simulink model "Demo_Kinect"  (R2014a)
settings: Solver=FixedStepDiscrete  SolverMode=SingleTasking  StartTime=0.0  StopTime=inf  FixedStep=0.01  RelTol=1e-3
PostLoadFcn:
  | h_RPStest = RPStest;
model workspace (MAT data in the model file):
  gtest = 0
undefined symbols (not defined in the file or in its folder): avert, avert_gaze_dirs_chance, avert_gaze_duration_factor, avert_head_frequency_factor, avert_head_speed, BML, BML1, BML2, bmlsL, bmlsM, bodyBusyFlag, clock, emotion_amount_factor, faceBusyFlag, fileID, GAZE_WIN, gazing, mutual_gaze_duration_factor, P, pose_chanc_factor, pose_chance_factor, pose_change_flag, pose_frequency_factor, pose_lean, pose_lean_flag, pose_selfAdaptor_chance_factor, pose_speed, pr, serial, STATE_BEFORE, STATE_GO, STATE_OVER, STATE_READY, Stateflow
libraries: simulink x22, instrumentlib x6, lib_affectiveChar_behavior x3, realtime_pacer_lib x2, lib_affectiveChar_input x1
(part 1 of 7)
CloseFcn:
  | % Try to close the GUI
  | % The user might have already closed it.
  | try
  | close(h_RPStest)
  | end
settings Model: ExtModeTrigDuration=2  Creator=Ulysses  LastModifiedBy=root180
settings OptimizationCC: OptimizeModelRefInitCode=on  LifeSpan=1
settings DebuggingCC: UnderspecifiedInitializationDetection=Classic  SolverPrmCheckMsg=none
settings HardwareCC: ProdBitPerInt=16  ProdBitPerPointer=8  ProdIntDivRoundTo=Zero  ProdEndianess=LittleEndian  ProdWordSize=8  ProdHWDeviceType=Atmel->AVR
settings RTWCC: SystemTargetFile=realtime.tlc  GenerateMakefile=off  TemplateMakefile=realtime.tmf  Description=Run on Target Hardware  RTWVerbose=off  ProcessScript=realtime_make_rtw_hook
settings STFCustomTargetCC: TargetLibSuffix=.a  GenerateSampleERTMain=on  ConcurrentExecutionCompliant=off  GeneratePreprocessorConditionals=Use local settings  ERTCustomFileBanners=on  SupportNonInlinedSFcns=off  SupportVariableSizeSignals=on  MATLABClassNameForMDSCustomization=Simulink.SoftwareTarget.ERTCustomization  GRTInterface=off  SystemTargetFile=realtime.tlc
settings ERTTargetCC: CombineOutputUpdateFcns=off  SupportContinuousTime=on  SupportVariableSizeSignals=on  ExtModeTransport=3  ExtModeMexFile=ext_serial_win32_comm  ExtModeMexArgs=0 1 9600  ERTSrcFileBannerTemplate=realtime_code_template.cgt  ERTHdrFileBannerTemplate=realtime_code_template.cgt  ERTDataSrcFileTemplate=realtime_code_template.cgt  ERTDataHdrFileTemplate=realtime_code_template.cgt  ERTCustomFileTemplate=realtime_file_process.tlc

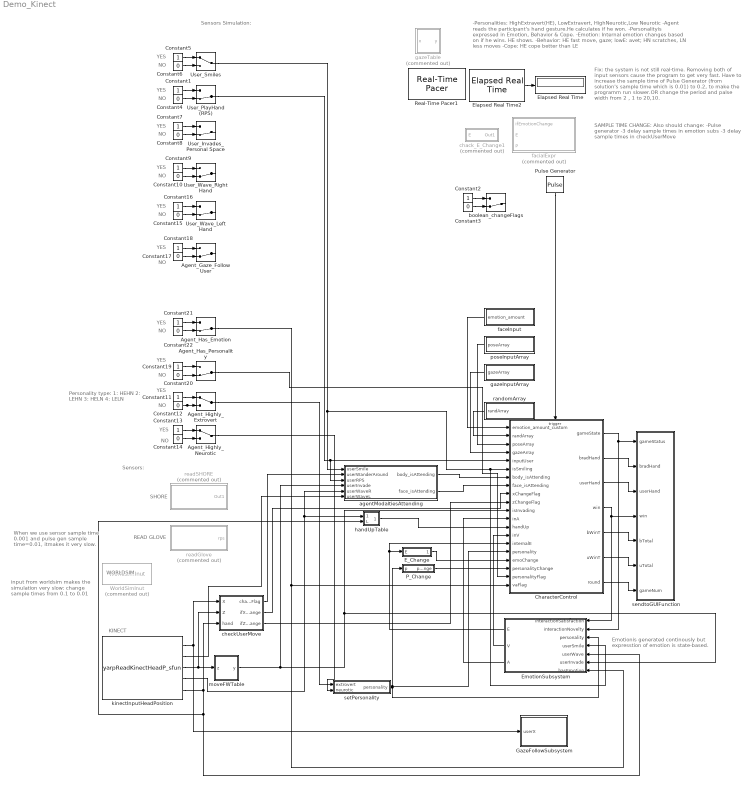
== system Demo_Kinect ==
  note: Sensors Simulation:
  note: YES
  note: YES
  note: Emotionis generated continously but expresstion of emotion is state-based.
  note: WORLDSIM
  note: SHORE
  note: READ GLOVE
  note: SAMPLE TIME CHANGE:
      | Also should change:
      | -Pulse generator
      | -3 delay sample times in emotion subs
      | -3 delay sample times in checkUserMove
  note: When we use sensor sample time 0.001 and pulse gen sample time=0.01, itmakes it very slow.
  note: input from worldsim makes the simulation very slow: change sample times from 0.1 to 0.01
  note: -Personalities: HighExtravert(HE), LowExtravert, HighNeurotic,Low Neurotic
      | -Agent reads the participant's hand gesture.He  calculates if he won.
      | -Personalityis expressed in Emotion, Behavior & Cope.
      | -Emotion: Internal emotion changes based on if he wins. HE shows.
      | -Behavior: HE fast move, gaze; lowE: avet; HN scratches, LN less moves
      | -Cope: HE cope better than LE
  note: Fix: the system is not still real-time. Removing both of input sensors cause the program to get very fast. Have to increase the sample time of Pulse Generator (from solution's sample time which is 0.01) to 0.2, to make the programm run slower.OR change the period and palse width from 2 , 1 to 20,10.
  note: YES
  note: YES
  note: YES
  note: YES
  note: YES
  note: NO
  note: NO
  note: NO
  note: NO
  note: NO
  note: NO
  note: NO
  note: YES
  note: NO
  note: Personality type:
      | 1: HEHN
      | 2: LEHN
      | 3: HELN
      | 4: LELN
  note: Sensors:
  note: KINECT
  note: YES
  note: NO
  note: YES
  note: NO
  Agent_Gaze_Follow User : ManualSwitch  CurrentSetting=0
  Agent_Has_Emotion : ManualSwitch  CurrentSetting=0
  Agent_Has_Personality : ManualSwitch  CurrentSetting=0
  Agent_Highly_Extrovert : ManualSwitch
  Agent_Highly_Neurotic : ManualSwitch
  CharacterControl : Stateflow chart  TreatAsAtomicUnit=on
  Constant{1,5,7,9,16,18} (6 alike) : Constant  OutDataTypeStr=double
  Constant{4,6,8,10,15,17} (6 alike) : Constant  Value=0  OutDataTypeStr=double
  Constant{2,11,13,19,21} (5 alike) : Constant  OutDataTypeStr=boolean
  Constant{3,12,14,20,22} (5 alike) : Constant  Value=0  OutDataTypeStr=boolean
  E_Change : Subsystem
  Elapsed Real Time : Display
      settings: Decimation=2
  Elapsed Real Time2 : realtime_pacer_lib/Elapsed Real Time
  EmotionSubsystem : Subsystem
  GazeFollowSubsystem : Subsystem
  P_Change : Subsystem
  Pulse Generator : DiscretePulseGenerator  SampleTime=0.01
  Real-Time Pacer1 : realtime_pacer_lib/Real-Time Pacer  simTimePerRealTime=1
  User_Invades_Personal Space : ManualSwitch  CurrentSetting=0
  User_PlayHand (RPS) : ManualSwitch  CurrentSetting=0
  User_Smiles : ManualSwitch
  User_Wave_Left Hand : ManualSwitch  CurrentSetting=0
  User_Wave_Right Hand : ManualSwitch  CurrentSetting=0
  WorldSimInut : lib_affectiveChar_input/WorldSimInut  Commented=on
  agentModaltiesAttending : Subsystem
  boolean_changeFlags : ManualSwitch  CurrentSetting=0
  chack_E_Change1 : Subsystem  Commented=on
  checkUserMove : Subsystem
  faceInput : Subsystem
  facialExpr : Subsystem  Commented=on
  gazeInputArray : Subsystem
  gazeTable : Truth Table  Commented=on  TreatAsAtomicUnit=on
  handUpTable : Truth Table  TreatAsAtomicUnit=on
  kinectInputHeadPosition : M-S-Function  FunctionName=yarpReadKinectHeadP_sfun  Parameters='/mary/output','/simulink/in0'
  moveFWTable : Truth Table  TreatAsAtomicUnit=on
  poseInputArray : Subsystem
  randomArray : Subsystem
  readGlove : Subsystem  Commented=on  AncestorBlock=lib_affectiveChar_input/readGlove
  readSHORE : Subsystem  Commented=on  AncestorBlock=lib_affectiveChar_input/readSHORE
  sendtoGUIFunction : MATLAB Function  TreatAsAtomicUnit=on
  setPersonality : MATLAB Function  TreatAsAtomicUnit=on
  wires:
  CharacterControl/1(gameState) -> EmotionSubsystem/2(interactionNovelty), sendtoGUIFunction/1(gameStatus)
  CharacterControl/2(bradHand) -> sendtoGUIFunction/2(bradHand)
  CharacterControl/3(userHand) -> sendtoGUIFunction/3(userHand)
  CharacterControl/6(uWinT) -> sendtoGUIFunction/6(uTotal)
  CharacterControl/7(round) -> sendtoGUIFunction/7(gameNum)
  kinectInputHeadPosition/3 -> moveFWTable/1(z), checkUserMove/2(Z)
  Elapsed Real Time2/1 -> Elapsed Real Time/1
  Pulse Generator/1 -> CharacterControl/Trigger
  CharacterControl/5(bWinT) -> sendtoGUIFunction/5(bTotal)
  CharacterControl/4(win) -> EmotionSubsystem/1(interactionSatisfaction), sendtoGUIFunction/4(win)
  kinectInputHeadPosition/5 -> handUpTable/2(L), EmotionSubsystem/5(userWave), checkUserMove/3(hand)
  kinectInputHeadPosition/1 -> checkUserMove/1(X), GazeFollowSubsystem/1(userX)
  randomArray/1(randArray) -> CharacterControl/2(randArray)
  EmotionSubsystem/1(E) -> CharacterControl/15(internalE), E_Change/1(E)
  EmotionSubsystem/2(V) -> CharacterControl/14(inV)
  EmotionSubsystem/3(A) -> CharacterControl/12(inA)
  E_Change/1(eChange) -> CharacterControl/17(emoChange)
  Constant8/1 -> User_Invades_Personal Space/2
  Constant7/1 -> User_Invades_Personal Space/1
  Constant10/1 -> User_Wave_Right Hand/2
  Constant9/1 -> User_Wave_Right Hand/1
  Constant12/1 -> Agent_Highly_Extrovert/2
  Constant11/1 -> Agent_Highly_Extrovert/1
  Constant14/1 -> Agent_Highly_Neurotic/2
  Constant13/1 -> Agent_Highly_Neurotic/1
  Agent_Highly_Extrovert/1 -> setPersonality/1(extrovert)
  Agent_Highly_Neurotic/1 -> setPersonality/2(neurotic)
  setPersonality/1(personality) -> EmotionSubsystem/3(personality), P_Change/1(p), CharacterControl/16(personality)
  Constant3/1 -> boolean_changeFlags/2
  Constant2/1 -> boolean_changeFlags/1
  Constant4/1 -> User_PlayHand (RPS)/2
  Constant1/1 -> User_PlayHand (RPS)/1
  Constant6/1 -> User_Smiles/2
  Constant5/1 -> User_Smiles/1
  User_PlayHand (RPS)/1 -> CharacterControl/5(inputUser), agentModaltiesAttending/3(userRPS)
  User_Smiles/1 -> agentModaltiesAttending/1(userSmile), CharacterControl/6(isSmiling), EmotionSubsystem/4(userSmile)
  P_Change/1(pChange) -> CharacterControl/18(personalityChange)
  Constant15/1 -> User_Wave_Left Hand/2
  Constant16/1 -> User_Wave_Left Hand/1
  Constant17/1 -> Agent_Gaze_Follow User/2
  Constant18/1 -> Agent_Gaze_Follow User/1
  gazeInputArray/1(gazeArray) -> CharacterControl/4(gazeArray)
  Constant19/1 -> Agent_Has_Personality/1
  Constant20/1 -> Agent_Has_Personality/2
  Constant21/1 -> Agent_Has_Emotion/1
  Constant22/1 -> Agent_Has_Emotion/2
  Agent_Has_Emotion/1 -> EmotionSubsystem/7(hasEmotion), CharacterControl/20(vaFlag)
  Agent_Has_Personality/1 -> CharacterControl/19(personalityFlag)
  poseInputArray/1(poseArray) -> CharacterControl/3(poseArray)
  faceInput/1(emotion_amount) -> CharacterControl/1(emotion_amount_custom)
  moveFWTable/1(y) -> agentModaltiesAttending/4(userInvade), EmotionSubsystem/6(userInvade), CharacterControl/11(isInvading)
  checkUserMove/2(ifXChange) -> CharacterControl/9(xChangeFlag)
  checkUserMove/3(ifZChange) -> CharacterControl/10(zChangeFlag)
  agentModaltiesAttending/1(body_isAttending) -> CharacterControl/7(body_isAttending)
  agentModaltiesAttending/2(face_isAttending) -> CharacterControl/8(face_isAttending)
  kinectInputHeadPosition/4 -> handUpTable/1(R), agentModaltiesAttending/5(userWaveR)
  kinectInputHeadPosition/2 -> agentModaltiesAttending/6(userWaveL)
  handUpTable/1(y) -> CharacterControl/13(handUp)
  checkUserMove/1(changeFlag) -> agentModaltiesAttending/2(userWanderAround)

== system Demo_Kinect/CharacterControl/Gaze_Controller ==
  randArray : Inport
  personality : Inport  Port=2
  inV : Inport  Port=3
  inA : Inport  Port=4
  personalityChange : Inport  Port=5
  gazeArray : Inport  Port=6
  secs : TriggerPort  ShowOutputPort=on
  " Demux " : Demux  Outputs=1
  " SFunction " : S-Function  Tag=Stateflow S-Function Demo_KinectWaveWalkInvade 9  FunctionName=sf_sfun  PortCounts=[7 2]  EnableBusSupport=off
  " Terminator " : Terminator
  gameState : Outport
  wires:
  randArray/1 -> " SFunction "/1
  personality/1 -> " SFunction "/2
  inV/1 -> " SFunction "/3
  inA/1 -> " SFunction "/4
  personalityChange/1 -> " SFunction "/5
  gazeArray/1 -> " SFunction "/6
  " SFunction "/2 -> gameState/1  "gameState"
  " Demux "/1 -> " Terminator "/1
  secs/1 -> " SFunction "/7
  " SFunction "/1 -> " Demux "/1

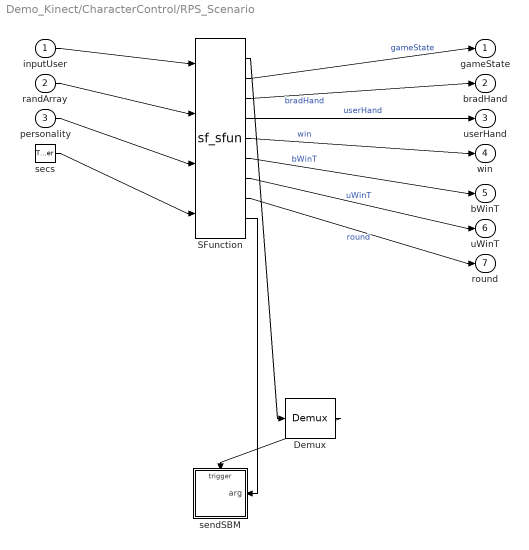
== system Demo_Kinect/CharacterControl/RPS_Scenario ==
  inputUser : Inport
  randArray : Inport  Port=2
  personality : Inport  Port=3
  secs : TriggerPort  ShowOutputPort=on
  " Demux " : Demux  Outputs=1
  " SFunction " : S-Function  Tag=Stateflow S-Function Demo_KinectWaveWalkInvade 5  FunctionName=sf_sfun  PortCounts=[4 9]  EnableBusSupport=off
  sendSBM : Subsystem
      settings: UndoDeleteFcn=Stateflow.SLINSF.SimulinkMan.restorePreDeleteFcn  PreDeleteFcn=Stateflow.SLINSF.SimulinkMan.removePreDeleteFcn
  gameState : Outport
  bradHand : Outport  Port=2
  userHand : Outport  Port=3
  win : Outport  Port=4
  bWinT : Outport  Port=5
  uWinT : Outport  Port=6
  round : Outport  Port=7
  wires:
  inputUser/1 -> " SFunction "/1
  randArray/1 -> " SFunction "/2
  personality/1 -> " SFunction "/3
  " SFunction "/2 -> gameState/1  "gameState"
  " SFunction "/3 -> bradHand/1  "bradHand"
  " SFunction "/4 -> userHand/1  "userHand"
  " SFunction "/5 -> win/1  "win"
  " SFunction "/6 -> bWinT/1  "bWinT"
  " SFunction "/7 -> uWinT/1  "uWinT"
  " SFunction "/8 -> round/1  "round"
  " SFunction "/9 -> sendSBM/1(arg)
  " Demux "/1 -> sendSBM/Trigger
  secs/1 -> " SFunction "/4
  " SFunction "/1 -> " Demux "/1

== system Demo_Kinect/CharacterControl/attention_Controller ==
  body_isAttending : Inport
  face_isAttending : Inport  Port=2
  secs : TriggerPort  ShowOutputPort=on
  " Demux " : Demux  Outputs=1
  " SFunction " : S-Function  Tag=Stateflow S-Function Demo_KinectWaveWalkInvade 10  FunctionName=sf_sfun  PortCounts=[3 1]  EnableBusSupport=off
  " Terminator " : Terminator
  wires:
  body_isAttending/1 -> " SFunction "/1
  face_isAttending/1 -> " SFunction "/2
  " Demux "/1 -> " Terminator "/1
  secs/1 -> " SFunction "/3
  " SFunction "/1 -> " Demux "/1

== system Demo_Kinect/CharacterControl/custom_Behavior_Factors ==
  inA : Inport
  inV : Inport  Port=2
  vaFlag : Inport  Port=3
  personalityFlag : Inport  Port=4
  gazeArray : Inport  Port=5
  personality : Inport  Port=6
  personalityChange : Inport  Port=7
  poseArray : Inport  Port=8
  emotion_amount_custom : Inport  Port=9
  " Demux " : Demux  Outputs=1
  " SFunction " : S-Function  Tag=Stateflow S-Function Demo_KinectWaveWalkInvade 44  FunctionName=sf_sfun  PortCounts=[9 1]  EnableBusSupport=off
  " Terminator " : Terminator
  sharedFunc : lib_affectiveChar_behavior/sharedFunc  SystemSampleTime=-1
  wires:
  inA/1 -> " SFunction "/1
  inV/1 -> " SFunction "/2
  vaFlag/1 -> " SFunction "/3
  personalityFlag/1 -> " SFunction "/4
  gazeArray/1 -> " SFunction "/5
  personality/1 -> " SFunction "/6
  personalityChange/1 -> " SFunction "/7
  poseArray/1 -> " SFunction "/8
  emotion_amount_custom/1 -> " SFunction "/9
  " Demux "/1 -> " Terminator "/1
  " SFunction "/1 -> " Demux "/1

== system Demo_Kinect/CharacterControl/emotion_Behavior_Factors ==
  inA : Inport
  inV : Inport  Port=2
  personality : Inport  Port=3
  gazeArray : Inport  Port=4
  emoChange : Inport  Port=5
  personalityFlag : Inport  Port=6
  vaFlag : Inport  Port=7
  poseArray : Inport  Port=8
  personalityChange : Inport  Port=9
  " Demux " : Demux  Outputs=1
  " SFunction " : S-Function  Tag=Stateflow S-Function Demo_KinectWaveWalkInvade 43  FunctionName=sf_sfun  PortCounts=[9 1]  EnableBusSupport=off
  " Terminator " : Terminator
  sharedFunc : lib_affectiveChar_behavior/sharedFunc  SystemSampleTime=-1
  wires:
  inA/1 -> " SFunction "/1
  inV/1 -> " SFunction "/2
  personality/1 -> " SFunction "/3
  gazeArray/1 -> " SFunction "/4
  emoChange/1 -> " SFunction "/5
  personalityFlag/1 -> " SFunction "/6
  vaFlag/1 -> " SFunction "/7
  poseArray/1 -> " SFunction "/8
  personalityChange/1 -> " SFunction "/9
  " Demux "/1 -> " Terminator "/1
  " SFunction "/1 -> " Demux "/1

== system Demo_Kinect/CharacterControl/facialExpression_Controller ==
  isSmiling : Inport
  personality : Inport  Port=2
  internalE : Inport  Port=3
  emoChange : Inport  Port=4
  emotion_amount_custom : Inport  Port=5
  secs : TriggerPort  ShowOutputPort=on
  " Demux " : Demux  Outputs=1
  " SFunction " : S-Function  Tag=Stateflow S-Function Demo_KinectWaveWalkInvade 11  FunctionName=sf_sfun  PortCounts=[6 2]  EnableBusSupport=off
  " Terminator " : Terminator
  gameState : Outport
  wires:
  isSmiling/1 -> " SFunction "/1
  personality/1 -> " SFunction "/2
  internalE/1 -> " SFunction "/3
  emoChange/1 -> " SFunction "/4
  emotion_amount_custom/1 -> " SFunction "/5
  " SFunction "/2 -> gameState/1  "gameState"
  " Demux "/1 -> " Terminator "/1
  secs/1 -> " SFunction "/6
  " SFunction "/1 -> " Demux "/1

== system Demo_Kinect/CharacterControl/idlePose_Controller ==
  inA : Inport
  inE : Inport  Port=2
  randArray : Inport  Port=3
  personality : Inport  Port=4
  inV : Inport  Port=5
  personalityChange : Inport  Port=6
  poseArray : Inport  Port=7
  secs : TriggerPort  ShowOutputPort=on
  " Demux " : Demux  Outputs=1
  " SFunction " : S-Function  Tag=Stateflow S-Function Demo_KinectWaveWalkInvade 4  FunctionName=sf_sfun  PortCounts=[8 2]  EnableBusSupport=off
  " Terminator " : Terminator
  gameState : Outport
  wires:
  inA/1 -> " SFunction "/1
  inE/1 -> " SFunction "/2
  randArray/1 -> " SFunction "/3
  personality/1 -> " SFunction "/4
  inV/1 -> " SFunction "/5
  personalityChange/1 -> " SFunction "/6
  poseArray/1 -> " SFunction "/7
  " SFunction "/2 -> gameState/1  "gameState"
  " Demux "/1 -> " Terminator "/1
  secs/1 -> " SFunction "/8
  " SFunction "/1 -> " Demux "/1

== system Demo_Kinect/CharacterControl/personalSpace_Controller ==
  distance : Inport
  zChange : Inport  Port=2
  secs : TriggerPort  ShowOutputPort=on
  " Demux " : Demux  Outputs=1
  " SFunction " : S-Function  Tag=Stateflow S-Function Demo_KinectWaveWalkInvade 8  FunctionName=sf_sfun  PortCounts=[3 2]  EnableBusSupport=off
  " Terminator " : Terminator
  gameState : Outport
  wires:
  distance/1 -> " SFunction "/1
  zChange/1 -> " SFunction "/2
  " SFunction "/2 -> gameState/1  "gameState"
  " Demux "/1 -> " Terminator "/1
  secs/1 -> " SFunction "/3
  " SFunction "/1 -> " Demux "/1

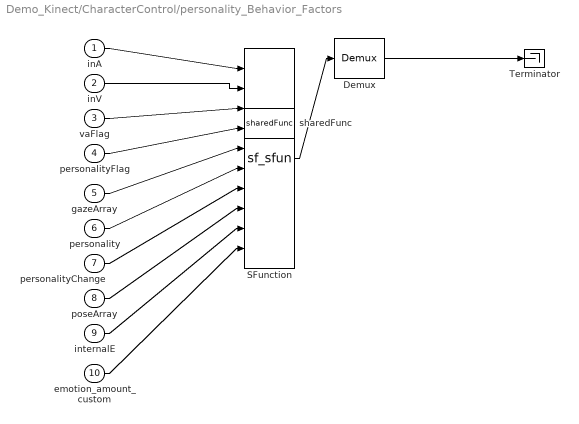
== system Demo_Kinect/CharacterControl/personality_Behavior_Factors ==
  inA : Inport
  inV : Inport  Port=2
  vaFlag : Inport  Port=3
  personalityFlag : Inport  Port=4
  gazeArray : Inport  Port=5
  personality : Inport  Port=6
  personalityChange : Inport  Port=7
  poseArray : Inport  Port=8
  internalE : Inport  Port=9
  emotion_amount_custom : Inport  Port=10
  " Demux " : Demux  Outputs=1
  " SFunction " : S-Function  Tag=Stateflow S-Function Demo_KinectWaveWalkInvade 42  FunctionName=sf_sfun  PortCounts=[10 1]  EnableBusSupport=off
  " Terminator " : Terminator
  sharedFunc : lib_affectiveChar_behavior/sharedFunc  SystemSampleTime=-1
  wires:
  inA/1 -> " SFunction "/1
  inV/1 -> " SFunction "/2
  vaFlag/1 -> " SFunction "/3
  personalityFlag/1 -> " SFunction "/4
  gazeArray/1 -> " SFunction "/5
  personality/1 -> " SFunction "/6
  personalityChange/1 -> " SFunction "/7
  poseArray/1 -> " SFunction "/8
  internalE/1 -> " SFunction "/9
  emotion_amount_custom/1 -> " SFunction "/10
  " Demux "/1 -> " Terminator "/1
  " SFunction "/1 -> " Demux "/1

== system Demo_Kinect/CharacterControl/sendBMLbyPriority.sendBML ==
  In1 : Inport  OutDataTypeStr=double  PortDimensions=[1000 1]
  f : TriggerPort  TriggerType=function-call
      settings: CopyFcn=Stateflow.SLINSF.SimulinkMan.removeBlockPreDeleteFcn  PreDeleteFcn=Stateflow.SLINSF.SimulinkMan.unsafePredeleteFcn
  C++ S-Function2 : S-Function  FunctionName=yarpSendText_sfun  Parameters='/sim/out/bml0', '/SB/in/bml'  EnableBusSupport=off
  wires:
  In1/1 -> C++ S-Function2/1

== system Demo_Kinect/CharacterControl/wave_Controller ==
  handUp : Inport
  personality : Inport  Port=2
  randArray : Inport  Port=3
  personalityChange : Inport  Port=4
  secs : TriggerPort  ShowOutputPort=on
  " Demux " : Demux  Outputs=1
  " SFunction " : S-Function  Tag=Stateflow S-Function Demo_KinectWaveWalkInvade 20  FunctionName=sf_sfun  PortCounts=[5 2]  EnableBusSupport=off
  " Terminator " : Terminator
  gameState : Outport
  wires:
  handUp/1 -> " SFunction "/1
  personality/1 -> " SFunction "/2
  randArray/1 -> " SFunction "/3
  personalityChange/1 -> " SFunction "/4
  " SFunction "/2 -> gameState/1  "gameState"
  " Demux "/1 -> " Terminator "/1
  secs/1 -> " SFunction "/5
  " SFunction "/1 -> " Demux "/1

== system Demo_Kinect/E_Change ==
  E : Inport
  Abs2 : Abs
  Compare To Constant2 : simulink/Logic and Bit Operations/Compare To Constant  relop=>  const=0.1  OutDataTypeStr=boolean
  Delay1 : Delay  DelayLength=1  InitialCondition=0  SampleTime=0.01
  Sum2 : Sum  Inputs=|+-
  eChange : Outport
  wires:
  E/1 -> Sum2/2, Delay1/1
  Delay1/1 -> Sum2/1
  Sum2/1 -> Abs2/1
  Abs2/1 -> Compare To Constant2/1
  Compare To Constant2/1 -> eChange/1

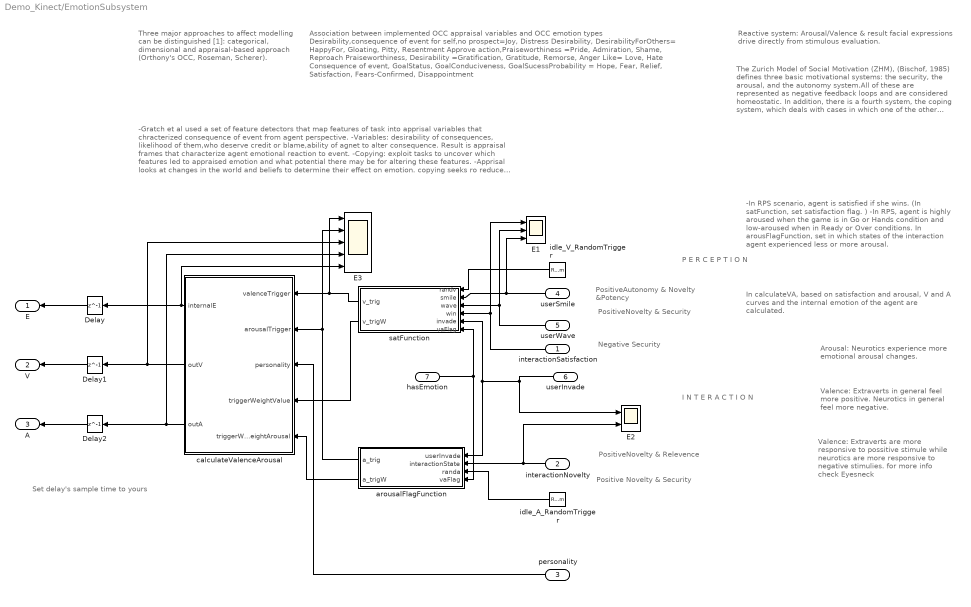
== system Demo_Kinect/EmotionSubsystem ==
  note: P
      | E
      | R
      | C
      | E
      | P
      | T
      | I
      | O
      | N
  note: PositiveNovelty &
      | Relevence
  note: The Zurich Model of Social Motivation (ZHM), (Bischof, 1985) defines three basic motivational systems: the security, the arousal, and the autonomy system.All of these are represented as negative feedback loops and are considered homeostatic. In addition, there is a fourth system, the coping system, which deals with cases in which one of the other systems gets blocked and cannot operate in its usual manner.( Bernardet and Schneider, 2013)
  note: PositiveNovelty &
      | Security
  note: Three major approaches to affect modelling can be distinguished [1]: categorical, dimensional and appraisal-based approach (Orthony's OCC, Roseman, Scherer).
  note: Reactive system: Arousal/Valence & result facial expressions drive directly from stimulous evaluation.
  note: Association between implemented OCC appraisal variables and OCC emotion types
      | Desirability,consequence of event for self,no prospect=Joy, Distress
      | Desirability, DesirabilityForOthers= HappyFor, Gloating, Pitty, Resentment
      | Approve action,Praiseworthiness =Pride, Admiration, Shame, Reproach
      | Praiseworthiness, Desirability =Gratification, Gratitude, Remorse, Anger
      | Like= Love, Hate
      | Consequence of event, GoalStatus, GoalConduciveness, GoalSucessProbability = Hope, Fear, Relief, Satisfaction, Fears-Confirmed, Disappointment
  note: -Gratch et al used a set of feature detectors that map features of task into apprisal variables that chracterized consequence of event from agent perspective.
      | -Variables: desirability of consequences, likelihood of them,who deserve credit or blame,ability of agnet to alter consequence. Result is appraisal frames that characterize agent emotional reaction to event.
      | -Copying: exploit tasks to uncover which features led to appraised emotion and what potential there may be for altering these features.
      | -Apprisal looks at changes in the world and beliefs to determine their effect on emotion.
      | copying seeks ro reduce (-) emotions by making changes to world or beliefs (problem-focused v.s. emotion-focused)
      | -For more info check Toward Virtual Humans, Swartout,w., et al (2006)
  note: In calculateVA, based on satisfaction and arousal, V and A curves and the internal emotion of the agent are calculated.
  note: Set delay's sample time to yours
  note: -In RPS scenario, agent is satisfied if she wins. (In satFunction, set satisfaction flag. )
      | -In RPS, agent is highly aroused when the game is in Go or Hands condition and low-aroused when in Ready or Over conditions.
      | In arousFlagFunction, set in which states of the interaction agent experienced less or more arousal.
  note: Valence: Extraverts are more responsive to possitive stimule while neurotics are more responsive to negative stimulies. for more info check Eyesneck
  note: Valence: Extraverts in general feel more positive. Neurotics in general feel more negative.
  note: Arousal: Neurotics experience more emotional arousal changes.
  note: Positive Novelty &
      | Security
  note: Negative Security
  note: PositiveAutonomy &
      | Novelty &Potency
  note: I
      | N
      | T
      | E
      | R
      | A
      | C
      | T
      | I
      | O
      | N
  interactionSatisfaction : Inport
  interactionNovelty : Inport  Port=2
  personality : Inport  Port=3
  userSmile : Inport  Port=4
  userWave : Inport  Port=5
  userInvade : Inport  Port=6
  hasEmotion : Inport  Port=7
  Delay : Delay  DelayLength=1  InitialCondition=0  SampleTime=0.01
  Delay1 : Delay  DelayLength=1  InitialCondition=0  SampleTime=0.01
  Delay2 : Delay  DelayLength=1  InitialCondition=0  SampleTime=0.01
  E1 : Scope  NumInputPorts=3
      settings: YMin=0.95~-20.15~-20.15  YMax=1.05~-19.15~-19.15  SaveName=ScopeData10
  E2 : Scope  NumInputPorts=2
      settings: TimeRange=10  YMin=-1~13.3  YMax=1~14.7  SaveName=ScopeData13
  E3 : Scope  NumInputPorts=5
      settings: TickLabels=on  YMin=-1~-1~-7.5~5~4  YMax=1~1~22.5~12~8  SaveName=ScopeData14  MaxDataPoints=10000
  arousalFlagFunction : MATLAB Function  TreatAsAtomicUnit=on
  calculateValenceArousal : Subsystem
  idle_A_RandomTrigger : UniformRandomNumber  Minimum=0  Maximum=100.9999  Seed=sum(10*clock)  SampleTime=0.1
  idle_V_RandomTrigger : UniformRandomNumber  Minimum=0  Maximum=100.9999  Seed=sum(10*clock)  SampleTime=0.1
  satFunction : MATLAB Function  TreatAsAtomicUnit=on
  E : Outport
  V : Outport  Port=2
  A : Outport  Port=3
  wires:
  calculateValenceArousal/1(internalE) -> E3/5, Delay/1
  Delay/1 -> E/1
  satFunction/1(v_trig) -> E3/1, calculateValenceArousal/1(valenceTrigger)
  arousalFlagFunction/1(a_trig) -> E3/2, calculateValenceArousal/2(arousalTrigger)
  calculateValenceArousal/2(outV) -> E3/3, Delay1/1
  calculateValenceArousal/3(outA) -> Delay2/1, E3/4
  Delay1/1 -> V/1
  Delay2/1 -> A/1
  personality/1 -> calculateValenceArousal/3(personality)
  interactionNovelty/1 -> arousalFlagFunction/2(interactionState), E2/2
  interactionSatisfaction/1 -> E1/1, satFunction/4(win)
  userInvade/1 -> arousalFlagFunction/1(userInvade), satFunction/5(invade), E2/1
  userSmile/1 -> E1/3, satFunction/2(smile)
  userWave/1 -> E1/2, satFunction/3(wave)
  idle_V_RandomTrigger/1 -> satFunction/1(randv)
  idle_A_RandomTrigger/1 -> arousalFlagFunction/3(randa)
  satFunction/2(v_trigW) -> calculateValenceArousal/4(triggerWeightValue)
  arousalFlagFunction/2(a_trigW) -> calculateValenceArousal/5(triggerWeightArousal)
  hasEmotion/1 -> satFunction/6(vaFlag), arousalFlagFunction/4(vaFlag)

== system Demo_Kinect/GazeFollowSubsystem ==
  note: Fix:since I'm activating the reactiveGaze module based on change in x,
      | it should be a change in ifUserChangeX (0-1 or 1-0) for it to be activated,
      | and if it is always 1 , ifuserchangex=1 then it does not activate.
  userX : Inport
  Y : Constant
  reactiveGaze : Subsystem
  wires:
  Y/1 -> reactiveGaze/2(y)
  userX/1 -> reactiveGaze/1(x)

== system Demo_Kinect/P_Change ==
  note: Problem: changing personality only changes the pChange value to 1 for 1 sample time which was very small and stateflow was not able to detect it.
      | Fix: Insreasing the sample time of the delay (10 times ,keeps the value 10 times, which is enough for pose subsystem to detect it and change the lean pose of agent.
  p : Inport
  Abs2 : Abs
  Compare To Constant2 : simulink/Logic and Bit Operations/Compare To Constant  relop=>  const=0.1  OutDataTypeStr=boolean
  Delay1 : Delay  DelayLength=1  InitialCondition=0  SampleTime=0.2
  Sum2 : Sum  Inputs=|+-
  pChange : Outport
  wires:
  Compare To Constant2/1 -> pChange/1
  Abs2/1 -> Compare To Constant2/1
  Sum2/1 -> Abs2/1
  Delay1/1 -> Sum2/1
  p/1 -> Delay1/1, Sum2/2

== system Demo_Kinect/agentModaltiesAttending ==
  note: Agent body idle can still generate BML but agent gaze idle should not.
  note: B
      | O
      | D
      | Y
  note: F
      | A
      | C
      | I
      | L
  note: Both agent body idle and agent gaze idle should not generate BML.
  userSmile : Inport
  userWanderAround : Inport  Port=2
  userRPS : Inport  Port=3
  userInvade : Inport  Port=4
  userWaveR : Inport  Port=5
  userWaveL : Inport  Port=6
  Logical Operator : Logic  Operator=OR  Inputs=4  AllPortsSameDT=off  OutDataTypeStr=boolean
  Logical Operator1 : Logic  Operator=OR  AllPortsSameDT=off  OutDataTypeStr=boolean
  body_isAttending : Outport
  face_isAttending : Outport  Port=2
  wires:
  Logical Operator/1 -> body_isAttending/1
  userInvade/1 -> Logical Operator/2
  userRPS/1 -> Logical Operator/1
  userWaveR/1 -> Logical Operator/3
  userWaveL/1 -> Logical Operator/4
  userSmile/1 -> Logical Operator1/1
  userWanderAround/1 -> Logical Operator1/2
  Logical Operator1/1 -> face_isAttending/1

== system Demo_Kinect/chack_E_Change1 ==
  E : Inport
  Scope : Scope  NumInputPorts=4
      settings: YMin=-1~-1~-1~6  YMax=1~1~1~6  SaveName=ScopeData9
  checkNeutral : MATLAB Function  TreatAsAtomicUnit=on
  eChange : Subsystem
  gaze : Logic  AllPortsSameDT=off  OutDataTypeStr=boolean
  Out1 : Outport
  wires:
  eChange/1(ifEChange) -> gaze/1, Scope/2
  gaze/1 -> Scope/1, Out1/1
  E/1 -> Scope/4, eChange/1(e), checkNeutral/1(e)
  checkNeutral/1(notNeutral) -> Scope/3, gaze/2

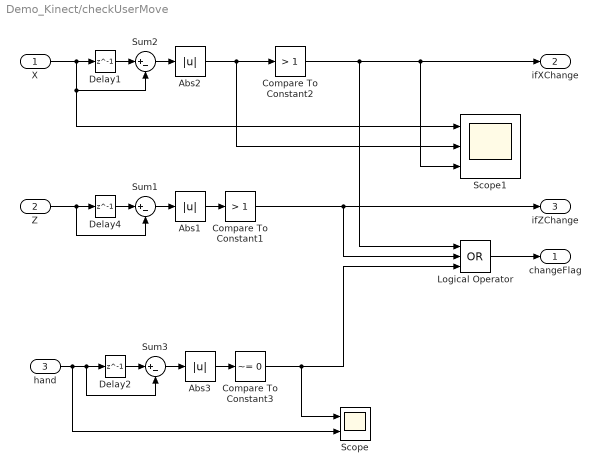
== system Demo_Kinect/checkUserMove ==
  X : Inport
  Z : Inport  Port=2
  hand : Inport  Port=3
  Abs1 : Abs
  Abs2 : Abs
  Abs3 : Abs
  Compare To Constant1 : simulink/Logic and Bit Operations/Compare To Constant  relop=>  const=1  OutDataTypeStr=boolean
  Compare To Constant2 : simulink/Logic and Bit Operations/Compare To Constant  relop=>  const=1  OutDataTypeStr=boolean
  Compare To Constant3 : simulink/Logic and Bit Operations/Compare To Constant  relop=~=  const=0  OutDataTypeStr=boolean
  Delay1 : Delay  DelayLength=1  InitialCondition=0  SampleTime=0.02
  Delay2 : Delay  DelayLength=1  InitialCondition=0  SampleTime=0.01
  Delay4 : Delay  DelayLength=1  InitialCondition=0  SampleTime=0.01
  Logical Operator : Logic  Operator=OR  Inputs=3  AllPortsSameDT=off  OutDataTypeStr=boolean
  Scope : Scope  NumInputPorts=2
      settings: YMin=-5~-5  YMax=5~5  SaveName=ScopeData4
  Scope1 : Scope  NumInputPorts=3
      settings: YMin=-77.8519~-5~-5  YMax=-77.8519~5~5  SaveName=ScopeData5
  Sum1 : Sum  Inputs=|+-
  Sum2 : Sum  Inputs=|+-
  Sum3 : Sum  Inputs=|+-
  changeFlag : Outport
  ifXChange : Outport  Port=2
  ifZChange : Outport  Port=3
  wires:
  Z/1 -> Sum1/2, Delay4/1
  Delay4/1 -> Sum1/1
  Sum1/1 -> Abs1/1
  Abs1/1 -> Compare To Constant1/1
  Compare To Constant1/1 -> Logical Operator/2, ifZChange/1
  X/1 -> Scope1/1, Sum2/2, Delay1/1
  Delay1/1 -> Sum2/1
  Sum2/1 -> Abs2/1
  Abs2/1 -> Scope1/2, Compare To Constant2/1
  Compare To Constant2/1 -> Logical Operator/1, Scope1/3, ifXChange/1
  hand/1 -> Scope/2, Sum3/2, Delay2/1
  Delay2/1 -> Sum3/1
  Sum3/1 -> Abs3/1
  Abs3/1 -> Compare To Constant3/1
  Compare To Constant3/1 -> Scope/1, Logical Operator/3
  Logical Operator/1 -> changeFlag/1

== system Demo_Kinect/faceInput ==
  emotion_amount_custom : Constant
  emotion_amount : Outport
  wires:
  emotion_amount_custom/1 -> emotion_amount/1

== system Demo_Kinect/facialExpr ==
  ifEmotionChange : Inport
  E : Inport  Port=2
  P : Inport  Port=3
  Scope : Scope  NumInputPorts=2
      settings: YMin=-1~6  YMax=1~6  SaveName=ScopeData2
  checkNeutral : MATLAB Function  TreatAsAtomicUnit=on
  facialExprGen : Subsystem
  gaze : Logic  AllPortsSameDT=off  OutDataTypeStr=boolean
  wires:
  checkNeutral/1(notNeutral) -> gaze/2
  gaze/1 -> facialExprGen/Trigger, Scope/1
  E/1 -> facialExprGen/1(e), Scope/2, checkNeutral/1(e)
  ifEmotionChange/1 -> gaze/1
  P/1 -> facialExprGen/2(p)

== system Demo_Kinect/gazeInputArray ==
  note: 1) if gaze_custom_flag=1, user controls the gaze variables (personality &emotion have no effect)
      | 2) mutual_gaze_duration_custom: default is 1 which gives btw 18-to-26; rangle=float e.g. 0.25 is mutDuration/4;  2 is mutDuration*2
      | 3) avert_gaze_duration_custom default is 1;same as mutual
      | 4) avert_head_frequency_custom default is 1, rangle=float values
      | 5) avert_head_speed_custom=if 1 normal, if 2 fast, if 3 slow
      | 6) avert_dirs_chance=if 1 chance of gaze-Up more, if 2 chance of gaze-Down more, otherwise normal
      | 			(dirChance==1) %extrovert %31 U, L & R, 6% D
      | 			(dirChance==2)%introvert  6% U, 64% D, %15 L & R
      | 			else normal total: 132 is 8 percent chance of not pure(UR,UL,DR,DL)
      | 				                 and 25 percent chance of pure(U,D,L,R)
  avert_gaze_duration_Custom : Constant  Value=0.001
  avert_head_frequency_Custom : Constant  Value=10
  avert_head_speed_custom : Constant  Value=3
  gaze_custom_flag : Constant  Value=0
  gaze_dir_Custom : Constant
  makeGazeArray : MATLAB Function  TreatAsAtomicUnit=on
  mutual_gaze_duration_Custom : Constant  Value=10
  gazeArray : Outport
  wires:
  makeGazeArray/1(y) -> gazeArray/1
  avert_head_frequency_Custom/1 -> makeGazeArray/4(r4)
  avert_gaze_duration_Custom/1 -> makeGazeArray/3(r3)
  mutual_gaze_duration_Custom/1 -> makeGazeArray/2(r2)
  avert_head_speed_custom/1 -> makeGazeArray/5(r5)
  gaze_custom_flag/1 -> makeGazeArray/1(r1)
  gaze_dir_Custom/1 -> makeGazeArray/6(r6)

== system Demo_Kinect/poseInputArray ==
  note: 1) if gaze_custom_flag=1, user controls the pose variables (personality &emotion have no effect)
      | 2) pose_selfAdaptor_chance_custom
      | 3) pose_chance_custom
      | 4) pose_frequency_custom
      | 5) pose_speed_custom
  makePoseArray : MATLAB Function  TreatAsAtomicUnit=on
  pose_chance_custom : Constant
  pose_custom_flag : Constant
  pose_frequency_custom : Constant
  pose_lean_custom : Constant
  pose_selfAdaptor_chance_custom : Constant
  pose_speed_custom : Constant
  poseArray : Outport
  wires:
  pose_custom_flag/1 -> makePoseArray/1(r1)
  pose_speed_custom/1 -> makePoseArray/5(r5)
  pose_frequency_custom/1 -> makePoseArray/4(r4)
  makePoseArray/1(y) -> poseArray/1
  pose_selfAdaptor_chance_custom/1 -> makePoseArray/2(r2)
  pose_chance_custom/1 -> makePoseArray/3(r3)
  pose_lean_custom/1 -> makePoseArray/6(r6)

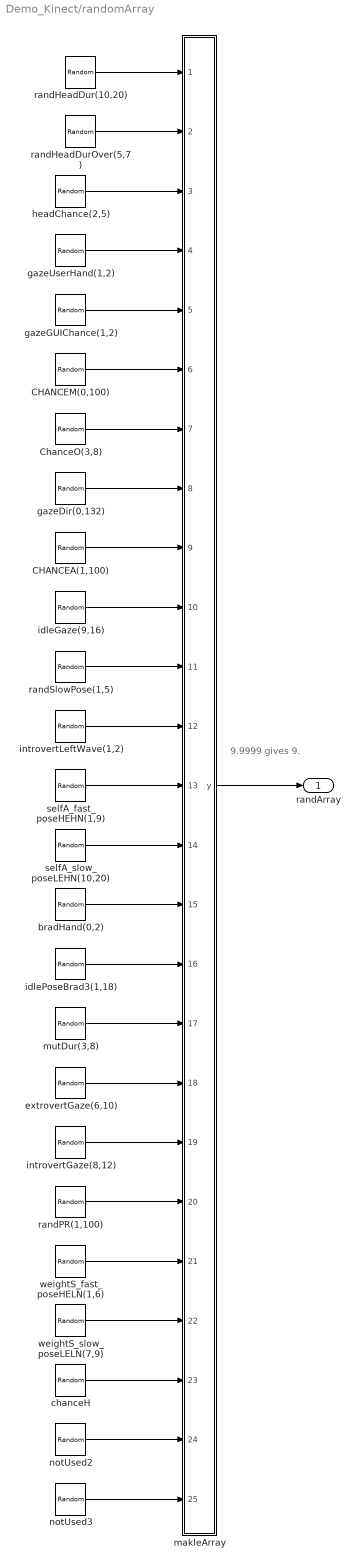
== system Demo_Kinect/randomArray ==
  note: 9.9999 gives 9.
  CHANCEA(1,100) : UniformRandomNumber  Minimum=1  Maximum=100.9999  Seed=sum(10*clock)  SampleTime=0.01
  CHANCEM(0,100) : UniformRandomNumber  Minimum=0  Maximum=100.9999  Seed=sum(10*clock)  SampleTime=0.01
  ChanceO(3,8) : UniformRandomNumber  Minimum=3  Maximum=8.9999  Seed=sum(10*clock)  SampleTime=0.01
  bradHand(0,2) : UniformRandomNumber  Minimum=0  Maximum=2.9999  Seed=sum(10*clock)  SampleTime=0.01
  chanceH : UniformRandomNumber  Minimum=8  Maximum=15.9999  Seed=sum(10*clock)  SampleTime=0.01
  extrovertGaze(6,10) : UniformRandomNumber  Minimum=6  Maximum=10.9999  Seed=sum(10*clock)  SampleTime=0.01
  gazeDir(0,132) : UniformRandomNumber  Minimum=0  Maximum=132.9999  Seed=sum(10*clock)  SampleTime=0.01
  gazeGUIChance(1,2) : UniformRandomNumber  Minimum=1  Maximum=2.9999  Seed=sum(10*clock)  SampleTime=0.01
  gazeUserHand(1,2) : UniformRandomNumber  Minimum=1  Maximum=2.9999  Seed=sum(10*clock)  SampleTime=0.01
  headChance(2,5) : UniformRandomNumber  Minimum=5  Maximum=10.9999  Seed=sum(10*clock)  SampleTime=0.01
  idleGaze(9,16) : UniformRandomNumber  Minimum=9  Maximum=16.9999  Seed=sum(10*clock)  SampleTime=0.01
  idlePoseBrad3(1,18) : UniformRandomNumber  Minimum=1  Maximum=18.9999  Seed=sum(10*clock)  SampleTime=0.01
  introvertGaze(8,12) : UniformRandomNumber  Minimum=8  Maximum=12.9999  Seed=sum(10*clock)  SampleTime=0.01
  introvertLeftWave(1,2) : UniformRandomNumber  Minimum=1  Maximum=2.9999  Seed=sum(10*clock)  SampleTime=0.01
  makleArray : MATLAB Function  TreatAsAtomicUnit=on
  mutDur(3,8) : UniformRandomNumber  Minimum=3  Maximum=8.9999  Seed=sum(10*clock)  SampleTime=0.01
  notUsed2 : UniformRandomNumber  Minimum=8  Maximum=12.9999  Seed=sum(10*clock)  SampleTime=0.01
  notUsed3 : UniformRandomNumber  Minimum=8  Maximum=12.9999  Seed=sum(10*clock)  SampleTime=0.01
  randHeadDur(10,20) : UniformRandomNumber  Minimum=10  Maximum=20.9999  Seed=sum(10*clock)  SampleTime=0.01
  randHeadDurOver(5,7) : UniformRandomNumber  Minimum=5  Maximum=7.9999  Seed=sum(10*clock)  SampleTime=0.01
  randPR(1,100) : UniformRandomNumber  Minimum=1  Maximum=100.9999  Seed=sum(10*clock)  SampleTime=0.01
  randSlowPose(1,5) : UniformRandomNumber  Minimum=1  Maximum=5.9999  Seed=sum(10*clock)  SampleTime=0.01
  selfA_fast_poseHEHN(1,9) : UniformRandomNumber  Minimum=1  Maximum=9.9999  Seed=sum(10*clock)  SampleTime=0.01
  selfA_slow_poseLEHN(10,20) : UniformRandomNumber  Minimum=10  Maximum=20.9999  Seed=sum(10*clock)  SampleTime=0.01
  weightS_fast_poseHELN(1,6) : UniformRandomNumber  Minimum=1  Maximum=6.9999  Seed=sum(10*clock)  SampleTime=0.01
  weightS_slow_poseLELN(7,9) : UniformRandomNumber  Minimum=7  Maximum=9.9999  Seed=sum(10*clock)  SampleTime=0.01
  randArray : Outport
  wires:
  randHeadDurOver(5,7)/1 -> makleArray/2(r2)
  makleArray/1(y) -> randArray/1
  gazeUserHand(1,2)/1 -> makleArray/4(r4)
  gazeGUIChance(1,2)/1 -> makleArray/5(r5)
  ChanceO(3,8)/1 -> makleArray/7(r7)
  randHeadDur(10,20)/1 -> makleArray/1(r1)
  headChance(2,5)/1 -> makleArray/3(r3)
  CHANCEM(0,100)/1 -> makleArray/6(r6)
  gazeDir(0,132)/1 -> makleArray/8(r8)
  CHANCEA(1,100)/1 -> makleArray/9(r9)
  idleGaze(9,16)/1 -> makleArray/10(r10)
  randSlowPose(1,5)/1 -> makleArray/11(r11)
  introvertLeftWave(1,2)/1 -> makleArray/12(r12)
  selfA_fast_poseHEHN(1,9)/1 -> makleArray/13(r13)
  selfA_slow_poseLEHN(10,20)/1 -> makleArray/14(r14)
  bradHand(0,2)/1 -> makleArray/15(r15)
  idlePoseBrad3(1,18)/1 -> makleArray/16(r16)
  mutDur(3,8)/1 -> makleArray/17(r17)
  extrovertGaze(6,10)/1 -> makleArray/18(r18)
  introvertGaze(8,12)/1 -> makleArray/19(r19)
  randPR(1,100)/1 -> makleArray/20(r20)
  weightS_fast_poseHELN(1,6)/1 -> makleArray/21(r21)
  weightS_slow_poseLELN(7,9)/1 -> makleArray/22(r22)
  chanceH/1 -> makleArray/23(r23)
  notUsed2/1 -> makleArray/24(r24)
  notUsed3/1 -> makleArray/25(r25)

== system Demo_Kinect/readGlove ==
  note: 1 paper
      | 0 scissors
      | 2 rock
  note: 0 paper
      | 1 scissors
      | 3 rock
  Subsystem : Subsystem  Commented=on
  convertFunction : MATLAB Function  TreatAsAtomicUnit=on
  normal glove : Subsystem
  rps : Outport
  wires:
  normal glove/1(Out1) -> convertFunction/1(u)
  convertFunction/1(y) -> rps/1

== system Demo_Kinect/readSHORE ==
  note: To remove the SHORE error if only value changes from 0 in one cycle ignore it.
  readSHORE : M-S-Function  FunctionName=yarpReadSHORE_sfun  Parameters='/testSender','/simulink/in'
  smile : Subsystem
  Out1 : Outport
  wires:
  smile/1(Out1) -> Out1/1
  readSHORE/1 -> smile/1(In1)

== system Demo_Kinect/CharacterControl/RPS_Scenario/sendSBM ==
  arg : Inport  OutDataTypeStr=double  PortDimensions=[256 1]
  f : TriggerPort  TriggerType=function-call
      settings: CopyFcn=Stateflow.SLINSF.SimulinkMan.removeBlockPreDeleteFcn  PreDeleteFcn=Stateflow.SLINSF.SimulinkMan.unsafePredeleteFcn
  C++ S-function2 : S-Function  FunctionName=yarpSendText_sfun  Parameters='/sim/out/smb0', '/SB/in/sbm'  EnableBusSupport=off
  wires:
  arg/1 -> C++ S-function2/1

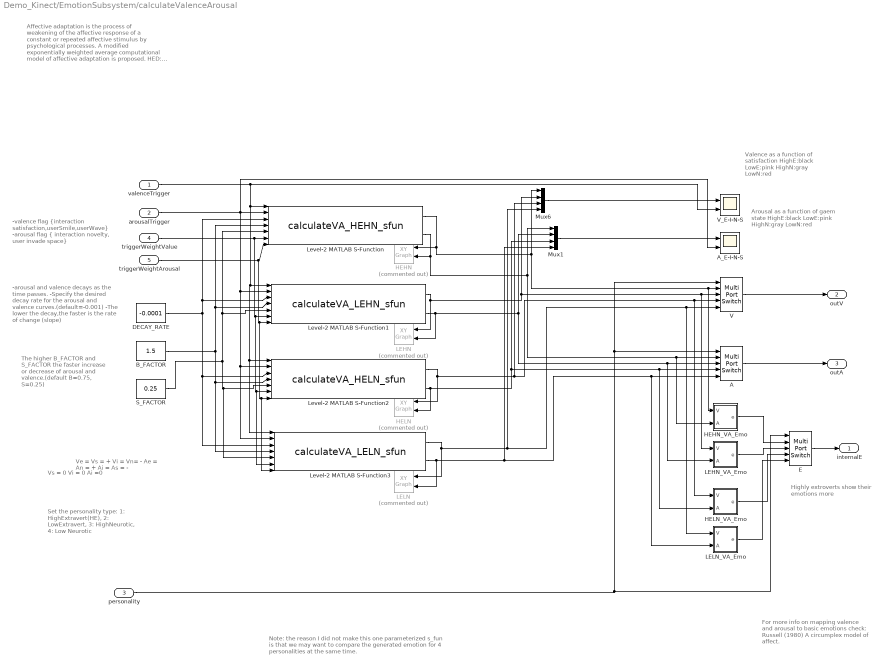
== system Demo_Kinect/EmotionSubsystem/calculateValenceArousal ==
  note: Highly extroverts show their emotions more
  note: Note: the reason I did not make this one parameterized s_fun is that we may want to compare the generated emotion for 4 personalities at the same time.
  note: For more info on mapping valence and arousal to basic emotions check: Russell (1980) A circumplex model of affect.
  note: Valence as a  function of satisfaction
      | HighE:black
      | LowE:pink
      | HighN:gray
      | LowN:red
  note: Set the personality type:
      | 1: HighExtravert(HE),
      | 2: LowExtravert,
      | 3: HighNeurotic,
      | 4: Low Neurotic
  note: The higher B_FACTOR and S_FACTOR the faster increase or decrease of arousal and valence.(default B=0.75, S=0.25)
  note: -arousal and valence decays as the time passes.
      | -Specify the desired decay rate for the arousal and valence curves.(default=-0.001)
      | -The lower the decay,the faster is the rate of change (slope)
  note: Vs = 0
      | Vi = 0
      | Ai =0
  note: Ve = Vs = +
      | Vi = Vn= -
      | Ae = An = +
      | Ai = As  = -
  note: Arousal as a function of gaem state
      | HighE:black
      | LowE:pink
      | HighN:gray
      | LowN:red
  note: Affective adaptation is the process of weakening of the affective response of a constant or repeated affective stimulus by psychological processes. A modified exponentially weighted average computational model of affective adaptation is proposed.
      |
      | HED: A Computational Model of Affective Adaptation and Emotion Dynamics, John E. Steephen
  note: -valence flag {interaction satisfaction,userSmile,userWave}
      | -arousal flag { interaction novelty, user invade space}
  valenceTrigger : Inport  OutDataTypeStr=double  PortDimensions=1
  arousalTrigger : Inport  Port=2  OutDataTypeStr=double  PortDimensions=1
  personality : Inport  Port=3  OutDataTypeStr=double  PortDimensions=1
  triggerWeightValue : Inport  Port=4  OutDataTypeStr=double  PortDimensions=1
  triggerWeightArousal : Inport  Port=5  OutDataTypeStr=double  PortDimensions=1
  A : MultiPortSwitch  Inputs=4
  A_E-I-N-S : Scope  NumInputPorts=2
      settings: YMin=-6~-1  YMax=5~1  SaveName=ScopeData11
  B_FACTOR : Constant  Value=1.5
  DECAY_RATE : Constant  Value=-0.0001
  E : MultiPortSwitch  Inputs=4
  HEHN : simulink/Sinks/XY Graph  Commented=on  xmin=-20  xmax=20  ymin=-20  ymax=20  st=-1
  HEHN_VA_Emo : Truth Table  TreatAsAtomicUnit=on
  HELN : simulink/Sinks/XY Graph  Commented=on  xmin=-20  xmax=20  ymin=-20  ymax=20  st=-1
  HELN_VA_Emo : Truth Table  TreatAsAtomicUnit=on
  LEHN : simulink/Sinks/XY Graph  Commented=on  xmin=-20  xmax=20  ymin=-20  ymax=20  st=-1
  LEHN_VA_Emo : Truth Table  TreatAsAtomicUnit=on
  LELN : simulink/Sinks/XY Graph  Commented=on  xmin=-20  xmax=20  ymin=-20  ymax=20  st=-1
  LELN_VA_Emo : Truth Table  TreatAsAtomicUnit=on
  Level-2 MATLAB S-Function : M-S-Function  FunctionName=calculateVA_HEHN_sfun
  Level-2 MATLAB S-Function1 : M-S-Function  FunctionName=calculateVA_LEHN_sfun
  Level-2 MATLAB S-Function2 : M-S-Function  FunctionName=calculateVA_HELN_sfun
  Level-2 MATLAB S-Function3 : M-S-Function  FunctionName=calculateVA_LELN_sfun
  Mux1 : Mux
  Mux6 : Mux
  S_FACTOR : Constant  Value=0.25
  V : MultiPortSwitch  Inputs=4
  V_E-I-N-S : Scope  NumInputPorts=2
      settings: TimeRange=10  YMin=-12~-1  YMax=10~1  SaveName=ScopeData6
  internalE : Outport
  outV : Outport  Port=2
  outA : Outport  Port=3
  wires:
  valenceTrigger/1 -> V_E-I-N-S/2, Level-2 MATLAB S-Function/1, Level-2 MATLAB S-Function3/1, Level-2 MATLAB S-Function2/1, Level-2 MATLAB S-Function1/1
  Level-2 MATLAB S-Function/2 -> HEHN/2, HEHN_VA_Emo/2(A), A/2, Mux1/1
  arousalTrigger/1 -> A_E-I-N-S/2, Level-2 MATLAB S-Function/2, Level-2 MATLAB S-Function3/2, Level-2 MATLAB S-Function2/2, Level-2 MATLAB S-Function1/2
  Level-2 MATLAB S-Function1/2 -> LEHN_VA_Emo/2(A), A/3, Mux1/2, LEHN/2
  Level-2 MATLAB S-Function/1 -> Mux6/1, HEHN_VA_Emo/1(V), V/2, HEHN/1
  Level-2 MATLAB S-Function1/1 -> Mux6/2, LEHN_VA_Emo/1(V), V/3, LEHN/1
  Level-2 MATLAB S-Function2/2 -> Mux1/3, HELN_VA_Emo/2(A), A/4, HELN/2
  Level-2 MATLAB S-Function3/2 -> LELN_VA_Emo/2(A), A/5, Mux1/4, LELN/2
  Level-2 MATLAB S-Function2/1 -> HELN_VA_Emo/1(V), V/4, Mux6/3, HELN/1
  Level-2 MATLAB S-Function3/1 -> LELN_VA_Emo/1(V), V/5, Mux6/4, LELN/1
  Mux1/1 -> A_E-I-N-S/1
  Mux6/1 -> V_E-I-N-S/1
  DECAY_RATE/1 -> Level-2 MATLAB S-Function/3, Level-2 MATLAB S-Function1/3, Level-2 MATLAB S-Function2/3, Level-2 MATLAB S-Function3/3
  B_FACTOR/1 -> Level-2 MATLAB S-Function/4, Level-2 MATLAB S-Function1/4, Level-2 MATLAB S-Function3/4, Level-2 MATLAB S-Function2/4
  S_FACTOR/1 -> Level-2 MATLAB S-Function3/5, Level-2 MATLAB S-Function2/5, Level-2 MATLAB S-Function1/5, Level-2 MATLAB S-Function/5
  V/1 -> outV/1
  A/1 -> outA/1
  personality/1 -> E/1, V/1, A/1
  triggerWeightValue/1 -> Level-2 MATLAB S-Function3/6, Level-2 MATLAB S-Function2/6, Level-2 MATLAB S-Function1/6, Level-2 MATLAB S-Function/6
  triggerWeightArousal/1 -> Level-2 MATLAB S-Function3/7, Level-2 MATLAB S-Function2/7, Level-2 MATLAB S-Function1/7, Level-2 MATLAB S-Function/7
  HEHN_VA_Emo/1(e) -> E/2
  LEHN_VA_Emo/1(e) -> E/3
  HELN_VA_Emo/1(e) -> E/4
  LELN_VA_Emo/1(e) -> E/5
  E/1 -> internalE/1

== system Demo_Kinect/GazeFollowSubsystem/reactiveGaze ==
  x : Inport
  y : Inport  Port=2
  createGazePawn : Stateflow chart  TreatAsAtomicUnit=on
  reactiveGazeControl : Subsystem
  wires:
  x/1 -> reactiveGazeControl/1(x)
  y/1 -> reactiveGazeControl/2(y)

== system Demo_Kinect/chack_E_Change1/eChange ==
  e : Inport
  Abs2 : Abs
  Compare To Constant2 : simulink/Logic and Bit Operations/Compare To Constant  relop=>  const=0.5  OutDataTypeStr=boolean
  Delay1 : Delay  DelayLength=1  InitialCondition=0  SampleTime=0.01
  Sum2 : Sum  Inputs=|+-
  ifEChange : Outport
  wires:
  e/1 -> Sum2/2, Delay1/1
  Delay1/1 -> Sum2/1
  Sum2/1 -> Abs2/1
  Abs2/1 -> Compare To Constant2/1
  Compare To Constant2/1 -> ifEChange/1

== system Demo_Kinect/facialExpr/facialExprGen ==
  e : Inport
  p : Inport  Port=2
  Trigger : TriggerPort  PortDimensions=1
  emotionBMLsLoop : Subsystem  Commented=on  TreatAsAtomicUnit=on
  forloop : Subsystem  Commented=on
  forloop1 : Subsystem
  matlabFuncIf : Subsystem
  setAU : MATLAB Function  TreatAsAtomicUnit=on
  setAmount : MATLAB Function  TreatAsAtomicUnit=on
  wires:
  p/1 -> setAmount/2(Pt)
  e/1 -> forloop1/4(e1), setAmount/1(E), setAU/1(E)
  setAU/1(AU) -> forloop1/2(AUs)
  setAmount/1(eAmountFactor) -> forloop1/1(Amounts)
  setAU/2(L) -> forloop1/3(L)

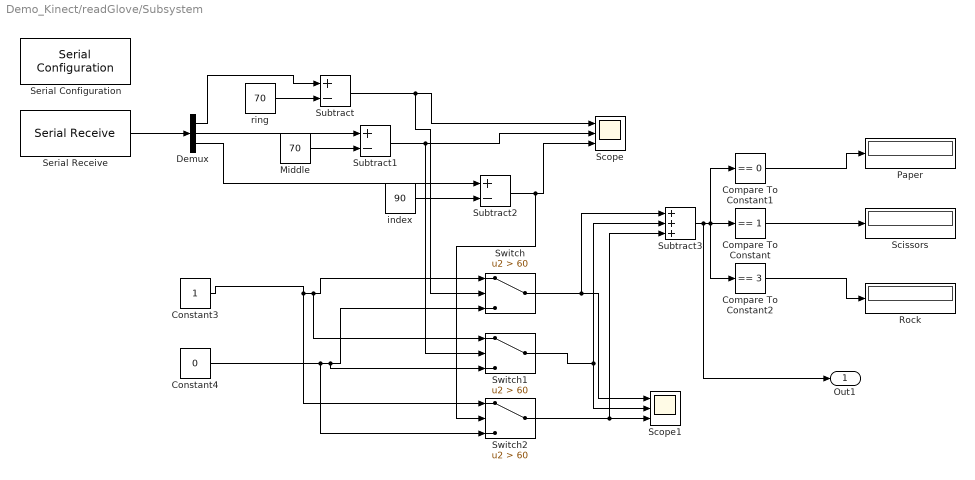
== system Demo_Kinect/readGlove/Subsystem ==
  Compare To Constant : simulink/Logic and Bit Operations/Compare To Constant  relop===  const=1  OutDataTypeStr=boolean
  Compare To Constant1 : simulink/Logic and Bit Operations/Compare To Constant  relop===  const=0  OutDataTypeStr=boolean
  Compare To Constant2 : simulink/Logic and Bit Operations/Compare To Constant  relop===  const=3  OutDataTypeStr=boolean
  Constant3 : Constant
  Constant4 : Constant  Value=0
  Demux : Demux  Outputs=3
  Middle : Constant  Value=70
  Paper : Display
  Rock : Display
  Scissors : Display
  Scope : Scope  NumInputPorts=3
      settings: YMin=-25~20~-25  YMax=200~200~200
  Scope1 : Scope  NumInputPorts=3
      settings: YMin=-0.5~-0.5~-1  YMax=1.5~1.5~1.5
  Serial Configuration : instrumentlib/Serial Configuration  Priority=-200000  ComPortMenu=COM4  ComPort=COM4  ObjConstructor=serial('COM4');  BaudRate=9600  DataBits=8  Parity=none  StopBits=1  FlowControl=none  Timeout=10  ByteOrder=LittleEndian
  Serial Receive : instrumentlib/Serial Receive  ComPortMenu=COM4  ComPort=COM4  ObjConstructor=serial('COM4');  Terminator=<none>  DataSize="[3  1]"  DataType=uint8  EnableBlockingMode=on  ActionDataUnavailable=Output last received value  CustomValue=0  SampleTime=0.01
  Subtract : Sum  Inputs=+-
  Subtract1 : Sum  Inputs=+-
  Subtract2 : Sum  Inputs=+-
  Subtract3 : Sum  Inputs=+++
  Switch : Switch  Criteria=u2 > Threshold  Threshold=60
  Switch1 : Switch  Criteria=u2 > Threshold  Threshold=60
  Switch2 : Switch  Criteria=u2 > Threshold  Threshold=60
  index : Constant  Value=90
  ring : Constant  Value=70
  Out1 : Outport
  wires:
  Demux/1 -> Subtract/1
  Demux/2 -> Subtract1/1
  Demux/3 -> Subtract2/1
  Subtract/1 -> Switch/2, Scope/1
  Subtract2/1 -> Switch2/2, Scope/3
  Subtract1/1 -> Switch1/2, Scope/2
  ring/1 -> Subtract/2
  Middle/1 -> Subtract1/2
  index/1 -> Subtract2/2
  Switch/1 -> Subtract3/1, Scope1/1
  Constant3/1 -> Switch2/1, Switch1/1, Switch/1
  Constant4/1 -> Switch2/3, Switch1/3, Switch/3
  Switch1/1 -> Subtract3/2, Scope1/2
  Switch2/1 -> Subtract3/3, Scope1/3
  Subtract3/1 -> Out1/1, Compare To Constant/1, Compare To Constant2/1, Compare To Constant1/1
  Compare To Constant1/1 -> Paper/1
  Compare To Constant/1 -> Scissors/1
  Compare To Constant2/1 -> Rock/1
  Serial Receive/1 -> Demux/1

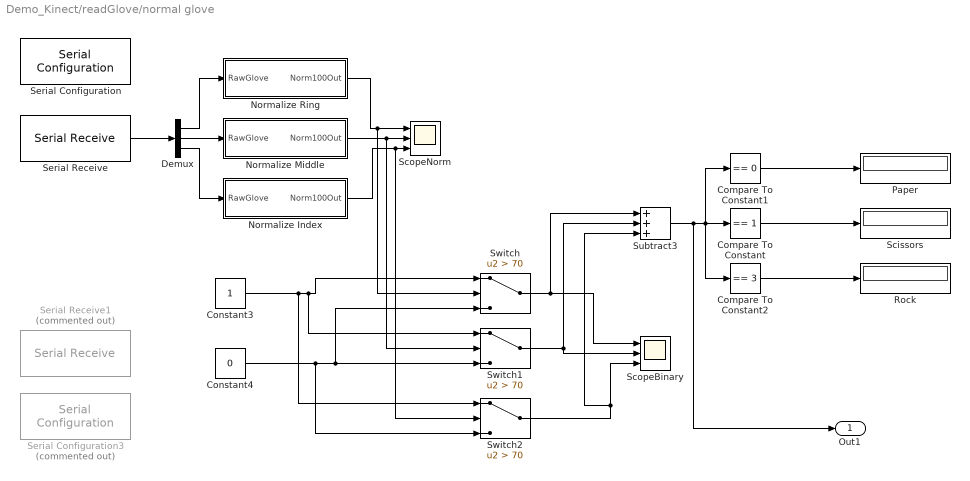
== system Demo_Kinect/readGlove/normal glove ==
  Compare To Constant : simulink/Logic and Bit Operations/Compare To Constant  relop===  const=1  OutDataTypeStr=boolean
  Compare To Constant1 : simulink/Logic and Bit Operations/Compare To Constant  relop===  const=0  OutDataTypeStr=boolean
  Compare To Constant2 : simulink/Logic and Bit Operations/Compare To Constant  relop===  const=3  OutDataTypeStr=boolean
  Constant3 : Constant
  Constant4 : Constant  Value=0
  Demux : Demux  Outputs=3
  Normalize Index : Subsystem
  Normalize Middle : Subsystem
  Normalize Ring : Subsystem
  Paper : Display
  Rock : Display
  Scissors : Display
  ScopeBinary : Scope  NumInputPorts=3
      settings: YMin=-0.5~-0.5~-0.5  YMax=1.5~1.5~1.5
  ScopeNorm : Scope  NumInputPorts=3
      settings: TimeRange=10  YMin=-20~-20~-20  YMax=150~150~150
  Serial Configuration : instrumentlib/Serial Configuration  Priority=-200000  ComPortMenu=COM4  ComPort=COM4  ObjConstructor=serial('COM4');  BaudRate=9600  DataBits=8  Parity=none  StopBits=1  FlowControl=none  Timeout=10  ByteOrder=LittleEndian
  Serial Configuration3 : instrumentlib/Serial Configuration  Priority=-200000  Commented=on  ComPortMenu=<Please select a port...>  ComPort=COM5  ObjConstructor=serial('COM5');  BaudRate=9600  DataBits=8  Parity=none  StopBits=1  FlowControl=none  Timeout=10  ByteOrder=LittleEndian
  Serial Receive : instrumentlib/Serial Receive  ComPortMenu=COM4  ComPort=COM4  ObjConstructor=serial('COM4');  Terminator=<none>  DataSize="[3  1]"  DataType=uint8  EnableBlockingMode=on  ActionDataUnavailable=Output last received value  CustomValue=0  SampleTime=0.01
  Serial Receive1 : instrumentlib/Serial Receive  Commented=on  ComPortMenu=<Please select a port...>  ComPort=COM5  ObjConstructor=serial('COM5');  Terminator=<none>  DataSize="[3  1]"  DataType=uint8  EnableBlockingMode=on  ActionDataUnavailable=Output last received value  CustomValue=0  SampleTime=0.01
  Subtract3 : Sum  Inputs=+++
  Switch : Switch  Criteria=u2 > Threshold  Threshold=70
  Switch1 : Switch  Criteria=u2 > Threshold  Threshold=70
  Switch2 : Switch  Criteria=u2 > Threshold  Threshold=70
  Out1 : Outport
  wires:
  Demux/1 -> Normalize Ring/1(RawGlove)
  Demux/2 -> Normalize Middle/1(RawGlove)
  Demux/3 -> Normalize Index/1(RawGlove)
  Switch/1 -> ScopeBinary/1, Subtract3/1
  Constant3/1 -> Switch2/1, Switch1/1, Switch/1
  Constant4/1 -> Switch2/3, Switch1/3, Switch/3
  Switch1/1 -> ScopeBinary/2, Subtract3/2
  Switch2/1 -> Subtract3/3, ScopeBinary/3
  Subtract3/1 -> Compare To Constant/1, Compare To Constant2/1, Compare To Constant1/1, Out1/1
  Compare To Constant1/1 -> Paper/1
  Compare To Constant/1 -> Scissors/1
  Compare To Constant2/1 -> Rock/1
  Normalize Index/1(Norm100Out) -> Switch2/2, ScopeNorm/3
  Normalize Ring/1(Norm100Out) -> Switch/2, ScopeNorm/1
  Normalize Middle/1(Norm100Out) -> ScopeNorm/2, Switch1/2
  Serial Receive/1 -> Demux/1

== system Demo_Kinect/readSHORE/smile ==
  In1 : Inport
  ifSmile : MATLAB Function  TreatAsAtomicUnit=on
  Out1 : Outport
  wires:
  ifSmile/1(y) -> Out1/1
  In1/1 -> ifSmile/1(u)

== system Demo_Kinect/GazeFollowSubsystem/reactiveGaze/createGazePawn/sendBML ==
  In1 : Inport  OutDataTypeStr=double  PortDimensions=[1000 1]
  f : TriggerPort  TriggerType=function-call
      settings: CopyFcn=Stateflow.SLINSF.SimulinkMan.removeBlockPreDeleteFcn  PreDeleteFcn=Stateflow.SLINSF.SimulinkMan.unsafePredeleteFcn
  C++ S-Function2 : S-Function  FunctionName=yarpSendText_sfun  Parameters='/sim/out/bml8', '/SB/in/bml'  EnableBusSupport=off
  wires:
  In1/1 -> C++ S-Function2/1
